simulink model "motor_model"  (R2022a)
settings: Solver=FixedStepAuto  StartTime=0.0  StopTime=sim_time  FixedStep=0.001  RelTol=1e-3
values from neighbouring files (symbols this model uses):
  den_c = C.den{:}    [main.m]
  den_sys = sys.den{:}    [main.m]
  Kd = pid_struct.Kd    [main.m]
  Ki = pid_struct.Ki    [main.m]
  Kp = pid_struct.Kp    [main.m]
  N = 1/pid_struct.Tf    [main.m]
  num_c = C.num{:}    [main.m]
  num_sys = sys.num{:}    [main.m]
libraries: simulink x1, slpidlib x1
settings Model: Creator=michi  LastModifiedBy=michi

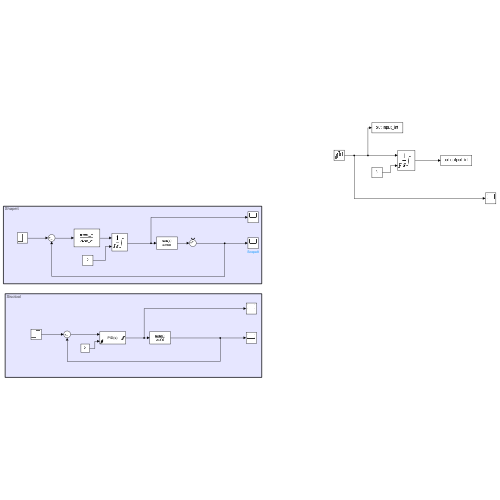
[thumbnail: Simulink's stored preview of the top-level diagram]
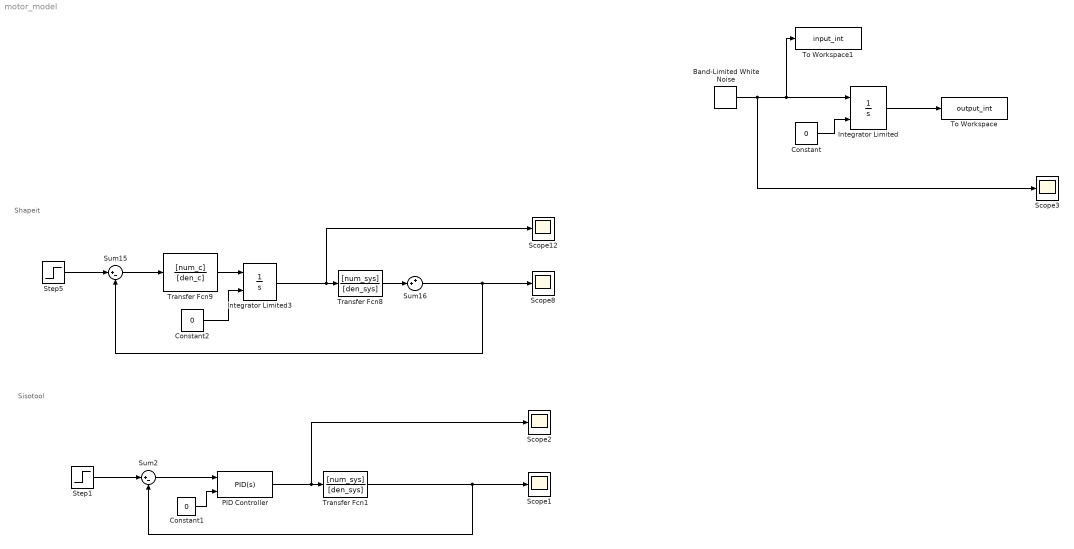
== system motor_model ==
  note: Sisotool
  note: Shapeit
  Band-Limited White Noise : simulink/Sources/Band-Limited White Noise  Cov=[1]  Ts=0.001  seed=[23341]
  Constant : Constant  Value=0
  Constant1 : Constant  Value=0
  Constant2 : Constant  Value=0
  Integrator Limited : Integrator  ExternalReset=rising  LimitOutput=on  UpperSaturationLimit=3  LowerSaturationLimit=-3
  Integrator Limited3 : Integrator  ExternalReset=rising  LimitOutput=on  UpperSaturationLimit=3  LowerSaturationLimit=-3
  PID Controller : slpidlib/PID Controller  Controller=PID  Form=Parallel  TimeDomain=Continuous-time  UseExternalTs=off  SampleTime=-1  IntegratorMethod=Forward Euler  FilterMethod=Forward Euler  ControllerParametersSource=internal  P=Kp  I=Ki  UseKiTs=off  D=Kd  N=N  UseFilter=on  TunerSelectOption=Transfer Function Based (PID Tuner App)  InitialConditionSource=internal  InitialConditionForIntegrator=0  InitialConditionForFilter=0  DifferentiatorICPrevScaledInput=0  ExternalReset=rising  TrackingMode=off  Kt=1  LimitOutput=on  SatLimitsSource=internal  UpperSaturationLimit=3  LowerSaturationLimit=-3  LinearizeAsGain=on  AntiWindupMode=none  Kb=1  POutMin=[]  POutMax=[]  IOutMin=[]  IOutMax=[]  DOutMin=[]  DOutMax=[]  NOutMin=[]  NOutMax=[]  SumOutMin=[]  SumOutMax=[]  SaturationOutMin=[]  SaturationOutMax=[]  PParamMin=[]  PParamMax=[]  IParamMin=[]  IParamMax=[]  DParamMin=[]  DParamMax=[]  NParamMin=[]  NParamMax=[]  KbParamMin=[]  KbParamMax=[]  KtParamMin=[]  KtParamMax=[]  KbOutMin=[]  KbOutMax=[]  KtOutMin=[]  KtOutMax=[]  IntegratorOutMin=[]  IntegratorOutMax=[]  FilterOutMin=[]  FilterOutMax=[]  SumI1OutMin=[]  SumI1OutMax=[]  SumI2OutMin=[]  SumI2OutMax=[]  SumI3OutMin=[]  SumI3OutMax=[]  SumI4OutMin=[]  SumI4OutMax=[]  SumDOutMin=[]  SumDOutMax=[]  DifferentiatorOutMin=[]  DifferentiatorOutMax=[]  FilterDiffOutCoefMin=[]  FilterDiffOutCoefMax=[]  ReciprocalOutMin=[]  ReciprocalOutMax=[]  SumDenOutMin=[]  SumDenOutMax=[]  SumNumOutMin=[]  SumNumOutMax=[]  DivideOutMin=[]  DivideOutMax=[]  UdiffTsProdOutMin=[]  UdiffTsProdOutMax=[]  NTsProdOutMin=[]  NTsProdOutMax=[]  UintegralTsProdOutMin=[]  UintegralTsProdOutMax=[]  UngainTsProdOutMin=[]  UngainTsProdOutMax=[]  IntegratorContinuousStateAttributes=''  IntegratorStateMustResolveToSignalObject=off  IntegratorRTWStateStorageClass=Auto  FilterContinuousStateAttributes=''  FilterStateMustResolveToSignalObject=off  FilterRTWStateStorageClass=Auto  ParallelPVariant=InternalParameters  IdealPVariant=Disabled  IVariant=InternalParameters  DVariant=InternalParameters  IntegratorVariant=Continuous  SatVariant=Enabled  AWVariant=Passthrough  PCopyVariant=Disabled  TRVariant=Disabled  FdbkBlocksVariant=Forward  IdealPFdbkVariant=Disabled  SatFdbkVariant=Disabled  DerivativeFilterVariant=ContFilter  NVariant=InternalParameters  NCopyVariant=Disabled  FilterICVariant=InternalICsFilter  IntegratorICVariant=InternalICs  ExternalResetVariant=ExternalReset  TRSumVariant=Passthrough  SumFdbkVariant=Disabled  SumVariant=Sum_PID  TsampFilterVariant=InternalTs  TsampNgainVariant=Passthrough  TsampIntegralVariant=Passthrough  ExternalSaturationOutDataTypeStr=Inherit: Same as second input  aMode=0
  Scope{1..3,8,12} (5 alike) : Scope
  Step1 : Step  After=0.03  SampleTime=0
  Step5 : Step  Time=2  SampleTime=0
  Sum15 : Sum  Inputs=|+-
  Sum16 : Sum  Inputs=++|
  Sum2 : Sum  Inputs=|+-
  To Workspace : ToWorkspace  VariableName=output_int  SampleTime=-1
  To Workspace1 : ToWorkspace  VariableName=input_int  SampleTime=-1
  Transfer Fcn1 : TransferFcn  Numerator=[num_sys]  Denominator=[den_sys]
  Transfer Fcn8 : TransferFcn  Numerator=[num_sys]  Denominator=[den_sys]
  Transfer Fcn9 : TransferFcn  Numerator=[num_c]  Denominator=[den_c]
  wires:
  Constant/1 -> Integrator Limited/2
  Band-Limited White Noise/1 -> Scope3/1, To Workspace1/1, Integrator Limited/1
  Integrator Limited/1 -> To Workspace/1
  Sum15/1 -> Transfer Fcn9/1
  Step5/1 -> Sum15/1
  Transfer Fcn8/1 -> Sum16/2
  Sum16/1 -> Scope8/1, Sum15/2
  Integrator Limited3/1 -> Scope12/1, Transfer Fcn8/1
  Transfer Fcn1/1 -> Scope1/1, Sum2/2
  Sum2/1 -> PID Controller/1
  Step1/1 -> Sum2/1
  Constant1/1 -> PID Controller/2
  Transfer Fcn9/1 -> Integrator Limited3/1
  Constant2/1 -> Integrator Limited3/2
  PID Controller/1 -> Scope2/1, Transfer Fcn1/1
